simulink model "rtdsa_example"  (R2016a)
settings: Solver=ode5  StartTime=0.0  StopTime=inf  FixedStep=0.001  RelTol=1e-3
undefined symbols (not defined in the file or in its folder): pow
libraries: simulink_extras x2
settings Model: SimulationMode=external  ExtModeArchiveMode=auto  ExtModeArchiveFileName=dsaData  ExtModeArchiveDirName=/Users/julianleland/Documents/Git/BitBucket/dcpctrl_v2/data/dsaData  ExtModeIncDirWhenArm=on  Creator=julianleland  LastModifiedBy=julianleland
settings DataIOCC: SaveOutput=off  SignalLogging=off  DSMLogging=off  SaveTime=off
settings HardwareCC: ProdBitPerLong=64  ProdLargestAtomicFloat=None  ProdHWDeviceType=Intel->x86-64  TargetBitPerLong=64  TargetBitPerPointer=64  TargetIntDivRoundTo=Zero  TargetEndianess=LittleEndian  TargetWordSize=64  TargetHWDeviceType=Intel->x86-64
settings RTWCC: SystemTargetFile=sldrt.tlc  TemplateMakefile=sldrt.tmf  Description=Simulink Desktop Real-Time  RTWCompilerOptimization=on
settings CodeAppCC: MaxIdLength=95
settings SimulinkDesktopRealTimeCC: TargetPreCompLibLocation=/Applications/MATLAB_R2016a.app/toolbox/sldrt/lib/maci64  TargetLangStandard=C89/C90 (ANSI)  SupportVariableSizeSignals=off

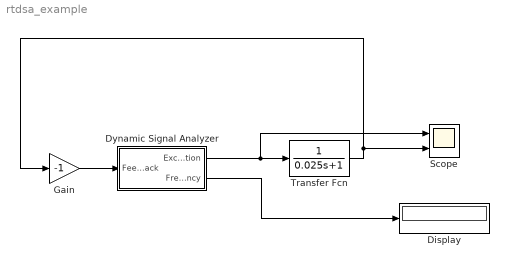
== system rtdsa_example ==
  Display : Display
  Dynamic Signal Analyzer : Subsystem  mask(AnalyzerBlock){analyzer_enable=on, aerrchk=1.0, avgcnt=3, winit=2*pi*50, wstop=2*pi*0.5, wmult=0.9, k_input=10, tsettle=0, Credits=Simulink Implementation : Marty Wand (1997-1998)}
      mask prompts: analyzer_enable "Enable"; aerrchk "Phase Angle Stability Criterion (degrees)"; avgcnt "# of Samples to Average per Frequency"; winit "Start Frequency (rad/sec)"; wstop "End Frequency (rad/sec)"; wmult "Frequency Multiplier"; k_input "Excitation Amplitude"; tsettle "Analyzer Start Time (sec)"
      mask help:
      | This subsystem simulates a dynamic system analyzer. The subsystem output is the swept sine Excitation signal and the subsystem input is the Feedback from the system being analyzed. The Frequency output can be connected to a display block to dynamically display the excitation frequency during simulation.
      |
      | The frequency response is stored in stack variable, freq_resp, as:
      |                            closed loop            open loop
      | freq(rad/sec)   gain   phase(deg)   gain   phase(deg)   time(sec)
      mask Help:
      | Credits:
      |   Original concept : Jim Royalty (1994)
      |   Original implementation : Jim Shouse (1995-1996)
      |   Enhanced implementation and ported to Simulink : Marty Wand (1997-1998)
      mask TypeOptions Credits: Simulink Implementation : Marty Wand (1997-1998) | Initial Concept : Jim Royalty (1994) | Proof of Concept : Jim Shouse (1995)
  Gain : Gain  Gain=-1
  Scope : Scope  NumInputPorts=2
  Transfer Fcn : TransferFcn  Denominator=[0.025 1]
  wires:
  Dynamic Signal Analyzer/1(Excitation) -> Scope/1, Transfer Fcn/1
  Transfer Fcn/1 -> Gain/1, Scope/2
  Gain/1 -> Dynamic Signal Analyzer/1(Feedback)
  Dynamic Signal Analyzer/2(Frequency) -> Display/1

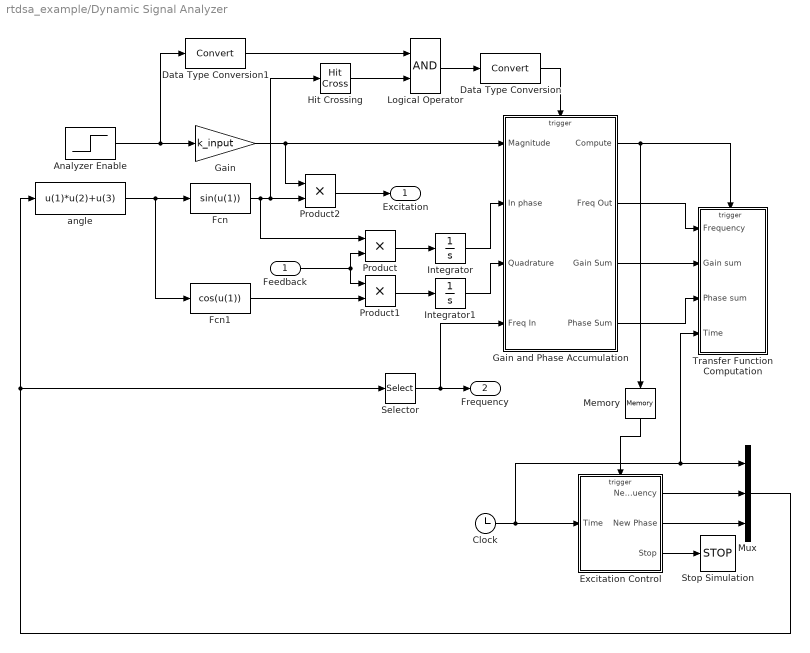
== system rtdsa_example/Dynamic Signal Analyzer ==
  Feedback : Inport
  Analyzer Enable : Step  Time=tsettle  After=analyzer_enable
  Clock : Clock
  Data Type Conversion : DataTypeConversion  SaturateOnIntegerOverflow=on  RndMeth=Zero
  Data Type Conversion1 : DataTypeConversion  SaturateOnIntegerOverflow=on  RndMeth=Zero
  Excitation Control : Subsystem  TreatAsAtomicUnit=on
  Fcn : Fcn  Expr=sin(u(1))
  Fcn1 : Fcn  Expr=cos(u(1))
  Gain : Gain  Gain=k_input  SaturateOnIntegerOverflow=on  OutDataTypeStr=Inherit: Same as input  ParamDataTypeStr=Inherit: Same as input
  Gain and Phase Accumulation : Subsystem  TreatAsAtomicUnit=on
  Hit Crossing : HitCross  HitCrossingDirection=rising
  Integrator : Integrator
  Integrator1 : Integrator
  Logical Operator : Logic
  Memory : Memory  InheritSampleTime=on
  Mux : Mux  Inputs=3
  Product : Product  SaturateOnIntegerOverflow=on  InputSameDT=on  OutDataTypeStr=Inherit: Same as first input
  Product1 : Product  SaturateOnIntegerOverflow=on  InputSameDT=on  OutDataTypeStr=Inherit: Same as first input
  Product2 : Product  SaturateOnIntegerOverflow=on  InputSameDT=on  OutDataTypeStr=Inherit: Same as first input
  Selector : Selector  InputPortWidth=3  IndexOptions=Index vector (dialog)  Indices=[2]  OutputSizes=1
  Stop Simulation : Stop
  Transfer Function Computation : Subsystem  TreatAsAtomicUnit=on
  angle : Fcn  Expr=u(1)*u(2)+u(3)
  Excitation : Outport  InitialOutput=0
  Frequency : Outport  Port=2  InitialOutput=0
  wires:
  Data Type Conversion1/1 -> Logical Operator/1
  Data Type Conversion/1 -> Gain and Phase Accumulation/Trigger
  angle/1 -> Fcn/1, Fcn1/1
  Product2/1 -> Excitation/1
  Fcn1/1 -> Product1/2
  Product/1 -> Integrator/1
  Product1/1 -> Integrator1/1
  Gain/1 -> Product2/1, Gain and Phase Accumulation/1(Magnitude)
  Logical Operator/1 -> Data Type Conversion/1
  Integrator/1 -> Gain and Phase Accumulation/2(In phase)
  Integrator1/1 -> Gain and Phase Accumulation/3(Quadrature)
  Gain and Phase Accumulation/4(Phase Sum) -> Transfer Function Computation/3(Phase sum)
  Gain and Phase Accumulation/3(Gain Sum) -> Transfer Function Computation/2(Gain sum)
  Gain and Phase Accumulation/2(Freq Out) -> Transfer Function Computation/1(Frequency)
  Excitation Control/3(Stop) -> Stop Simulation/1
  Clock/1 -> Excitation Control/1(Time), Mux/1, Transfer Function Computation/4(Time)
  Excitation Control/2(New Phase) -> Mux/3
  Mux/1 -> angle/1, Selector/1
  Fcn/1 -> Hit Crossing/1, Product2/2, Product/1
  Feedback/1 -> Product1/1, Product/2
  Hit Crossing/1 -> Logical Operator/2
  Analyzer Enable/1 -> Data Type Conversion1/1, Gain/1
  Excitation Control/1(New Frequency) -> Mux/2
  Selector/1 -> Frequency/1, Gain and Phase Accumulation/4(Freq In)
  Gain and Phase Accumulation/1(Compute) -> Transfer Function Computation/Trigger, Memory/1
  Memory/1 -> Excitation Control/Trigger

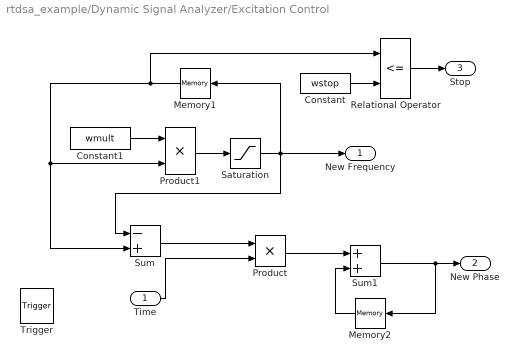
== system rtdsa_example/Dynamic Signal Analyzer/Excitation Control ==
  Time : Inport
  Trigger : TriggerPort  VariantControl=Variant
  Constant : Constant  Value=wstop
  Constant1 : Constant  Value=wmult
  Memory1 : Memory  X0=winit  InheritSampleTime=on
  Memory2 : Memory  InheritSampleTime=on
  Product : Product  SaturateOnIntegerOverflow=on  InputSameDT=on  OutDataTypeStr=Inherit: Same as first input
  Product1 : Product  SaturateOnIntegerOverflow=on  InputSameDT=on  OutDataTypeStr=Inherit: Same as first input
  Relational Operator : RelationalOperator  Operator=<=  InputSameDT=on
  Saturation : Saturate  UpperLimit=winit  LowerLimit=wstop
  Sum : Sum  Inputs=-+  SaturateOnIntegerOverflow=on  InputSameDT=on  OutDataTypeStr=Inherit: Same as first input
  Sum1 : Sum  SaturateOnIntegerOverflow=on  InputSameDT=on  OutDataTypeStr=Inherit: Same as first input
  New Frequency : Outport  InitialOutput=winit
  New Phase : Outport  Port=2  InitialOutput=0
  Stop : Outport  Port=3  InitialOutput=0
  wires:
  Product1/1 -> Saturation/1
  Time/1 -> Product/2
  Product/1 -> Sum1/1
  Constant1/1 -> Product1/1
  Sum/1 -> Product/1
  Sum1/1 -> New Phase/1, Memory2/1
  Memory2/1 -> Sum1/2
  Saturation/1 -> Sum/1, Memory1/1, New Frequency/1
  Constant/1 -> Relational Operator/2
  Relational Operator/1 -> Stop/1
  Memory1/1 -> Product1/2, Sum/2, Relational Operator/1

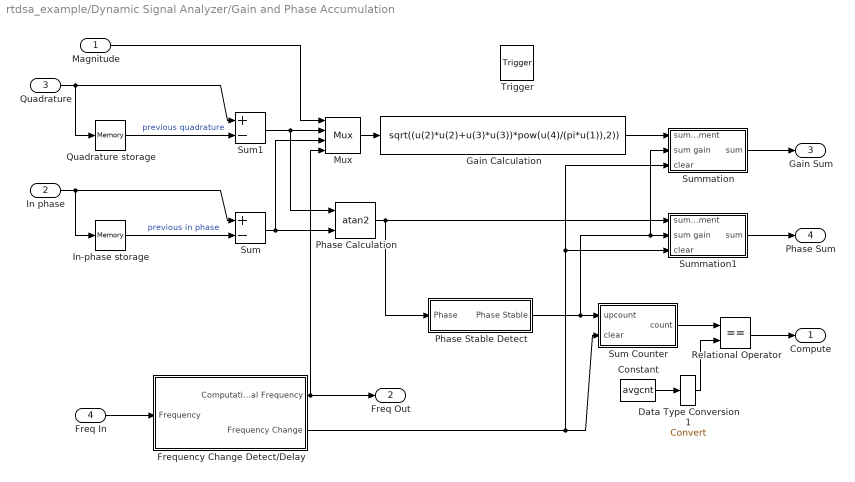
== system rtdsa_example/Dynamic Signal Analyzer/Gain and Phase Accumulation ==
  Magnitude : Inport
  In phase : Inport  Port=2
  Quadrature : Inport  Port=3
  Freq In : Inport  Port=4
  Trigger : TriggerPort  VariantControl=Variant
  Constant : Constant  Value=avgcnt
  Data Type Conversion1 : DataTypeConversion  SaturateOnIntegerOverflow=on  RndMeth=Zero
  Frequency Change Detect/Delay : Subsystem
  Gain Calculation : Fcn  Expr=sqrt((u(2)*u(2)+u(3)*u(3))*pow(u(4)/(pi*u(1)),2))
  In-phase storage : Memory  InheritSampleTime=on
  Mux : Mux
  Phase Calculation : Trigonometry  Operator=atan2
  Phase Stable Detect : Subsystem
  Quadrature storage : Memory  InheritSampleTime=on
  Relational Operator : RelationalOperator  Operator===  InputSameDT=on
  Sum : Sum  Inputs=+-  SaturateOnIntegerOverflow=on  InputSameDT=on  OutDataTypeStr=Inherit: Same as first input
  Sum Counter : Subsystem
  Sum1 : Sum  Inputs=+-  SaturateOnIntegerOverflow=on  InputSameDT=on  OutDataTypeStr=Inherit: Same as first input
  Summation : Subsystem
  Summation1 : Subsystem
  Compute : Outport  InitialOutput=0
  Freq Out : Outport  Port=2  InitialOutput=winit
  Gain Sum : Outport  Port=3  InitialOutput=0
  Phase Sum : Outport  Port=4  InitialOutput=0
  wires:
  Data Type Conversion1/1 -> Relational Operator/2
  Mux/1 -> Gain Calculation/1
  In-phase storage/1 -> Sum/2  "previous in phase"
  In phase/1 -> Sum/1, In-phase storage/1
  Quadrature storage/1 -> Sum1/2  "previous quadrature"
  Quadrature/1 -> Sum1/1, Quadrature storage/1
  Sum1/1 -> Mux/2, Phase Calculation/1
  Sum/1 -> Mux/3, Phase Calculation/2
  Magnitude/1 -> Mux/1
  Phase Stable Detect/1(Phase Stable) -> Sum Counter/1(upcount), Summation/2(sum gain), Summation1/2(sum gain)
  Frequency Change Detect/Delay/2(Frequency Change) -> Sum Counter/2(clear), Summation/3(clear), Summation1/3(clear)
  Frequency Change Detect/Delay/1(Computational Frequency) -> Mux/4, Freq Out/1
  Freq In/1 -> Frequency Change Detect/Delay/1(Frequency)
  Phase Calculation/1 -> Phase Stable Detect/1(Phase), Summation1/1(sum increment)
  Relational Operator/1 -> Compute/1
  Summation1/1(sum) -> Phase Sum/1
  Summation/1(sum) -> Gain Sum/1
  Gain Calculation/1 -> Summation/1(sum increment)
  Constant/1 -> Data Type Conversion1/1
  Sum Counter/1(count) -> Relational Operator/1

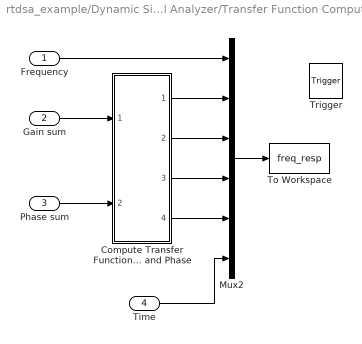
== system rtdsa_example/Dynamic Signal Analyzer/Transfer Function Computation ==
  Frequency : Inport
  Gain sum : Inport  Port=2
  Phase sum : Inport  Port=3
  Time : Inport  Port=4
  Trigger : TriggerPort  VariantControl=Variant
  Compute Transfer Function Gain and Phase : Subsystem
  Mux2 : Mux  Inputs=6
  To Workspace : ToWorkspace  VariableName=freq_resp  SampleTime=-1
  wires:
  Frequency/1 -> Mux2/1
  Mux2/1 -> To Workspace/1
  Compute Transfer Function Gain and Phase/4(OL phase) -> Mux2/5
  Compute Transfer Function Gain and Phase/3(OL gain) -> Mux2/4
  Compute Transfer Function Gain and Phase/2(CL phase) -> Mux2/3
  Compute Transfer Function Gain and Phase/1(CL gain) -> Mux2/2
  Gain sum/1 -> Compute Transfer Function Gain and Phase/1(Gain Sum)
  Phase sum/1 -> Compute Transfer Function Gain and Phase/2(Phase Sum)
  Time/1 -> Mux2/6

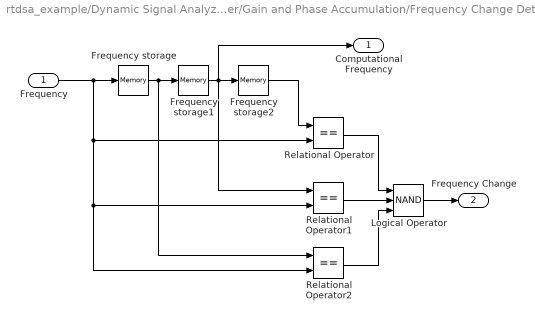
== system rtdsa_example/Dynamic Signal Analyzer/Gain and Phase Accumulation/Frequency Change Detect//Delay ==
  Frequency : Inport
  Frequency storage : Memory  X0=1e-6  InheritSampleTime=on
  Frequency storage1 : Memory  X0=1e-6  InheritSampleTime=on
  Frequency storage2 : Memory  X0=1e-6  InheritSampleTime=on
  Logical Operator : Logic  Operator=NAND  Inputs=3
  Relational Operator : RelationalOperator  Operator===  InputSameDT=on
  Relational Operator1 : RelationalOperator  Operator===  InputSameDT=on
  Relational Operator2 : RelationalOperator  Operator===  InputSameDT=on
  Computational Frequency : Outport  InitialOutput=0
  Frequency Change : Outport  Port=2  InitialOutput=0
  wires:
  Logical Operator/1 -> Frequency Change/1
  Frequency storage/1 -> Frequency storage1/1, Relational Operator2/1
  Relational Operator/1 -> Logical Operator/1
  Relational Operator1/1 -> Logical Operator/2
  Relational Operator2/1 -> Logical Operator/3
  Frequency/1 -> Frequency storage/1, Relational Operator/2, Relational Operator1/2, Relational Operator2/2
  Frequency storage2/1 -> Relational Operator/1
  Frequency storage1/1 -> Frequency storage2/1, Relational Operator1/1, Computational Frequency/1

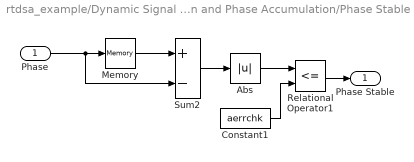
== system rtdsa_example/Dynamic Signal Analyzer/Gain and Phase Accumulation/Phase Stable Detect ==
  Phase : Inport
  Abs : Abs  SaturateOnIntegerOverflow=on
  Constant1 : Constant  Value=aerrchk
  Memory : Memory  X0=1e20  InheritSampleTime=on
  Relational Operator1 : RelationalOperator  Operator=<=  InputSameDT=on
  Sum2 : Sum  Inputs=+-  SaturateOnIntegerOverflow=on  InputSameDT=on  OutDataTypeStr=Inherit: Same as first input
  Phase Stable : Outport  InitialOutput=0
  wires:
  Phase/1 -> Memory/1, Sum2/2
  Sum2/1 -> Abs/1
  Constant1/1 -> Relational Operator1/2
  Abs/1 -> Relational Operator1/1
  Memory/1 -> Sum2/1
  Relational Operator1/1 -> Phase Stable/1

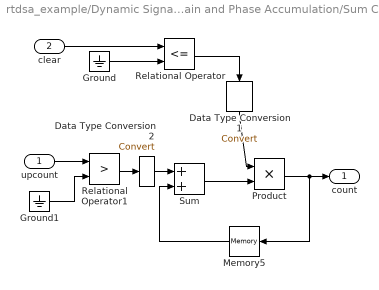
== system rtdsa_example/Dynamic Signal Analyzer/Gain and Phase Accumulation/Sum Counter ==
  upcount : Inport
  clear : Inport  Port=2
  Data Type Conversion1 : DataTypeConversion  SaturateOnIntegerOverflow=on  RndMeth=Zero
  Data Type Conversion2 : DataTypeConversion  SaturateOnIntegerOverflow=on  RndMeth=Zero
  Ground : Ground
  Ground1 : Ground
  Memory5 : Memory  InheritSampleTime=on
  Product : Product  SaturateOnIntegerOverflow=on  InputSameDT=on  OutDataTypeStr=Inherit: Same as first input
  Relational Operator : RelationalOperator  Operator=<=  InputSameDT=on
  Relational Operator1 : RelationalOperator  Operator=>  InputSameDT=on
  Sum : Sum  SaturateOnIntegerOverflow=on  InputSameDT=on  OutDataTypeStr=Inherit: Same as first input
  count : Outport
  wires:
  Data Type Conversion2/1 -> Sum/1
  Data Type Conversion1/1 -> Product/1
  Memory5/1 -> Sum/2
  Sum/1 -> Product/2
  Product/1 -> count/1, Memory5/1
  clear/1 -> Relational Operator/1
  Ground/1 -> Relational Operator/2
  Relational Operator/1 -> Data Type Conversion1/1
  upcount/1 -> Relational Operator1/1
  Relational Operator1/1 -> Data Type Conversion2/1
  Ground1/1 -> Relational Operator1/2

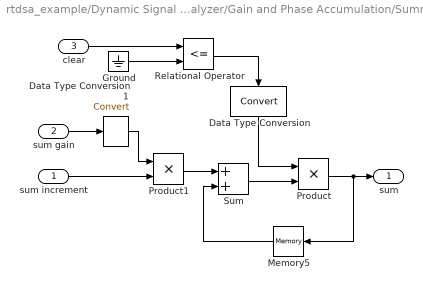
== system rtdsa_example/Dynamic Signal Analyzer/Gain and Phase Accumulation/Summation ==
  sum increment : Inport
  sum gain : Inport  Port=2
  clear : Inport  Port=3
  Data Type Conversion : DataTypeConversion  SaturateOnIntegerOverflow=on  RndMeth=Zero
  Data Type Conversion1 : DataTypeConversion  SaturateOnIntegerOverflow=on  RndMeth=Zero
  Ground : Ground
  Memory5 : Memory  InheritSampleTime=on
  Product : Product  SaturateOnIntegerOverflow=on  InputSameDT=on  OutDataTypeStr=Inherit: Same as first input
  Product1 : Product  SaturateOnIntegerOverflow=on  InputSameDT=on  OutDataTypeStr=Inherit: Same as first input
  Relational Operator : RelationalOperator  Operator=<=  InputSameDT=on
  Sum : Sum  SaturateOnIntegerOverflow=on  InputSameDT=on  OutDataTypeStr=Inherit: Same as first input
  sum : Outport
  wires:
  Data Type Conversion1/1 -> Product1/1
  Data Type Conversion/1 -> Product/1
  Product/1 -> Memory5/1, sum/1
  Sum/1 -> Product/2
  Memory5/1 -> Sum/2
  Relational Operator/1 -> Data Type Conversion/1
  Ground/1 -> Relational Operator/2
  clear/1 -> Relational Operator/1
  Product1/1 -> Sum/1
  sum increment/1 -> Product1/2
  sum gain/1 -> Data Type Conversion1/1

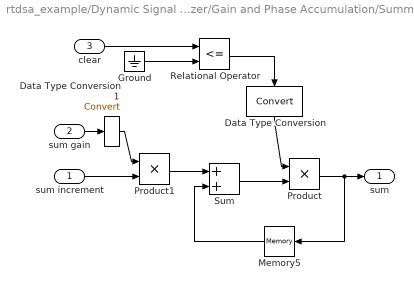
== system rtdsa_example/Dynamic Signal Analyzer/Gain and Phase Accumulation/Summation1 ==
  sum increment : Inport
  sum gain : Inport  Port=2
  clear : Inport  Port=3
  Data Type Conversion : DataTypeConversion  SaturateOnIntegerOverflow=on  RndMeth=Zero
  Data Type Conversion1 : DataTypeConversion  SaturateOnIntegerOverflow=on  RndMeth=Zero
  Ground : Ground
  Memory5 : Memory  InheritSampleTime=on
  Product : Product  SaturateOnIntegerOverflow=on  InputSameDT=on  OutDataTypeStr=Inherit: Same as first input
  Product1 : Product  SaturateOnIntegerOverflow=on  InputSameDT=on  OutDataTypeStr=Inherit: Same as first input
  Relational Operator : RelationalOperator  Operator=<=  InputSameDT=on
  Sum : Sum  SaturateOnIntegerOverflow=on  InputSameDT=on  OutDataTypeStr=Inherit: Same as first input
  sum : Outport
  wires:
  Data Type Conversion1/1 -> Product1/1
  Data Type Conversion/1 -> Product/1
  sum gain/1 -> Data Type Conversion1/1
  sum increment/1 -> Product1/2
  Product1/1 -> Sum/1
  clear/1 -> Relational Operator/1
  Ground/1 -> Relational Operator/2
  Relational Operator/1 -> Data Type Conversion/1
  Memory5/1 -> Sum/2
  Sum/1 -> Product/2
  Product/1 -> sum/1, Memory5/1

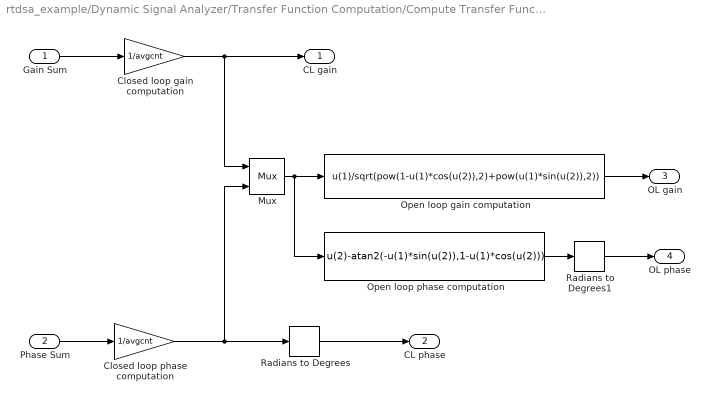
== system rtdsa_example/Dynamic Signal Analyzer/Transfer Function Computation/Compute Transfer Function Gain and Phase ==
  Gain Sum : Inport
  Phase Sum : Inport  Port=2
  Closed loop gain computation : Gain  Gain=1/avgcnt  SaturateOnIntegerOverflow=on  OutDataTypeStr=Inherit: Same as input  ParamDataTypeStr=Inherit: Same as input
  Closed loop phase computation : Gain  Gain=1/avgcnt  SaturateOnIntegerOverflow=on  OutDataTypeStr=Inherit: Same as input  ParamDataTypeStr=Inherit: Same as input
  Mux : Mux  Inputs=2
  Open loop gain computation : Fcn  Expr=u(1)/sqrt(pow(1-u(1)*cos(u(2)),2)+pow(u(1)*sin(u(2)),2))
  Open loop phase computation : Fcn  Expr=u(2)-atan2(-u(1)*sin(u(2)),1-u(1)*cos(u(2)))
  Radians to Degrees : simulink_extras/Transformations/Radians to Degrees
  Radians to Degrees1 : simulink_extras/Transformations/Radians to Degrees
  CL gain : Outport  InitialOutput=0
  CL phase : Outport  Port=2  InitialOutput=0
  OL gain : Outport  Port=3  InitialOutput=0
  OL phase : Outport  Port=4  InitialOutput=0
  wires:
  Open loop gain computation/1 -> OL gain/1
  Mux/1 -> Open loop gain computation/1, Open loop phase computation/1
  Radians to Degrees/1 -> CL phase/1
  Radians to Degrees1/1 -> OL phase/1
  Open loop phase computation/1 -> Radians to Degrees1/1
  Phase Sum/1 -> Closed loop phase computation/1
  Closed loop phase computation/1 -> Mux/2, Radians to Degrees/1
  Gain Sum/1 -> Closed loop gain computation/1
  Closed loop gain computation/1 -> CL gain/1, Mux/1
